simulink model "lab5_2"  (R2020b)
settings: Solver=VariableStepAuto  StartTime=0.0  StopTime=60  RelTol=1e-3
model workspace (MAT data in the model file):
  Kf = 100
  Kp = 100
  x = Simulink.Parameter
  x.Value = 0
  x.DataType = 'auto'
  x.Dimensions = [1 1]
  y = Simulink.Parameter
  y.Value = 1
  y.DataType = 'auto'
  y.Dimensions = [1 1]
settings Model: Creator=Dexp  LastModifiedBy=takem

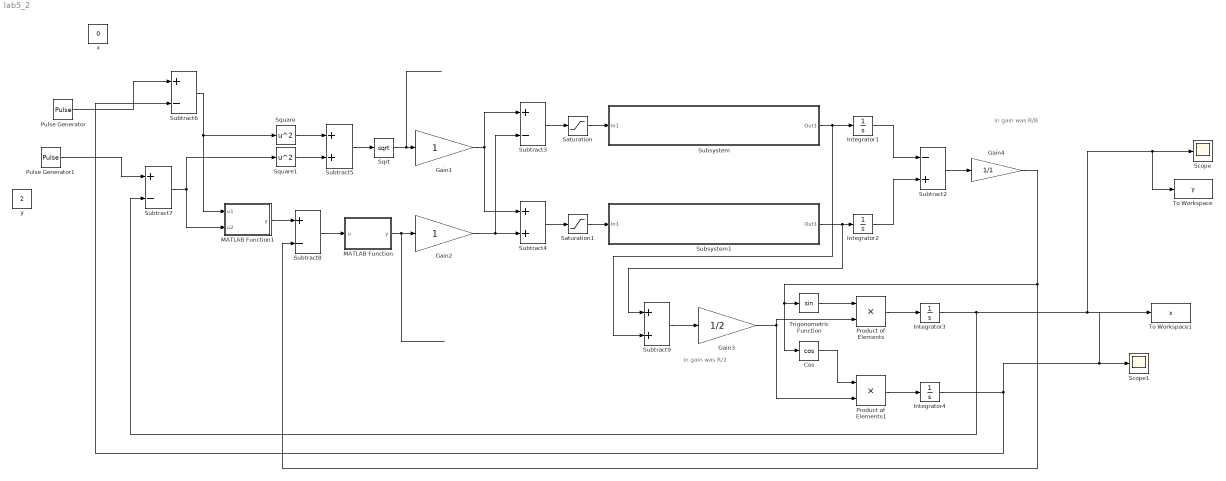
== system lab5_2 ==
  note: in gain was
      | R/B
  note: in gain was
      | R/2
  Cos : Trigonometry  Operator=cos
  Gain1 : Gain
  Gain2 : Gain
  Gain3 : Gain  Gain=1/2
  Gain4 : Gain  Gain=1/1
  Integrator{1..4} (4 alike) : Integrator
  MATLAB Function : MATLAB Function  TreatAsAtomicUnit=on
  MATLAB Function1 : MATLAB Function  TreatAsAtomicUnit=on
  Product of Elements : Product  Inputs=**
  Product of Elements1 : Product  Inputs=**
  Pulse Generator : DiscretePulseGenerator  PulseType=Time based  Period=60  PulseWidth=5  PhaseDelay=30
  Pulse Generator1 : DiscretePulseGenerator  PulseType=Time based  Amplitude=0.5  Period=60  PulseWidth=5  PhaseDelay=60  VectorParams1D=off
  Saturation : Saturate  UpperLimit=100  LowerLimit=-100
  Saturation1 : Saturate  UpperLimit=100  LowerLimit=-100
  Scope : Scope
  Scope1 : Scope
  Sqrt : Sqrt  SaturateOnIntegerOverflow=on
  Square : Math  Operator=square  SaturateOnIntegerOverflow=on
  Square1 : Math  Operator=square  SaturateOnIntegerOverflow=on
  Subsystem : Subsystem
  Subsystem1 : Subsystem
  Subtract2 : Sum  Inputs=-+
  Subtract{3,6..8} (4 alike) : Sum  Inputs=+-
  Subtract4 : Sum
  Subtract5 : Sum
  Subtract9 : Sum
  To Workspace : ToWorkspace  VariableName=y  SampleTime=-1
  To Workspace1 : ToWorkspace  VariableName=x  SampleTime=-1
  Trigonometric Function : Trigonometry
  x : Constant  Value=0
  y : Constant  Value=2
  wires:
  Integrator1/1 -> Subtract2/1
  Saturation/1 -> Subsystem/1(In1)
  Subsystem/1(Out1) -> Subtract9/2, Integrator1/1
  Subsystem1/1(Out1) -> Subtract9/1, Integrator2/1
  Integrator2/1 -> Subtract2/2
  Subtract2/1 -> Gain4/1
  Saturation1/1 -> Subsystem1/1(In1)
  Subtract3/1 -> Saturation/1
  Subtract4/1 -> Saturation1/1
  Subtract5/1 -> Sqrt/1
  Sqrt/1 -> Gain1/1
  Gain1/1 -> Subtract3/1, Subtract4/1
  Gain2/1 -> Subtract3/2, Subtract4/2
  Square/1 -> Subtract5/1
  Square1/1 -> Subtract5/2
  MATLAB Function/1(y) -> Gain2/1
  Subtract8/1 -> MATLAB Function/1(u)
  MATLAB Function1/1(y) -> Subtract8/1
  Subtract6/1 -> MATLAB Function1/1(u1), Square/1
  Subtract7/1 -> MATLAB Function1/2(u2), Square1/1
  Subtract9/1 -> Gain3/1
  Gain4/1 -> Cos/1, Trigonometric Function/1, Subtract8/2
  Trigonometric Function/1 -> Product of Elements/1
  Cos/1 -> Product of Elements1/1
  Gain3/1 -> Product of Elements/2, Product of Elements1/2
  Product of Elements1/1 -> Integrator4/1
  Product of Elements/1 -> Integrator3/1
  Integrator3/1 -> Subtract7/2, To Workspace/1, Scope/1
  Integrator4/1 -> To Workspace1/1, Scope1/1, Subtract6/2
  Pulse Generator/1 -> Subtract6/1
  Pulse Generator1/1 -> Subtract7/1

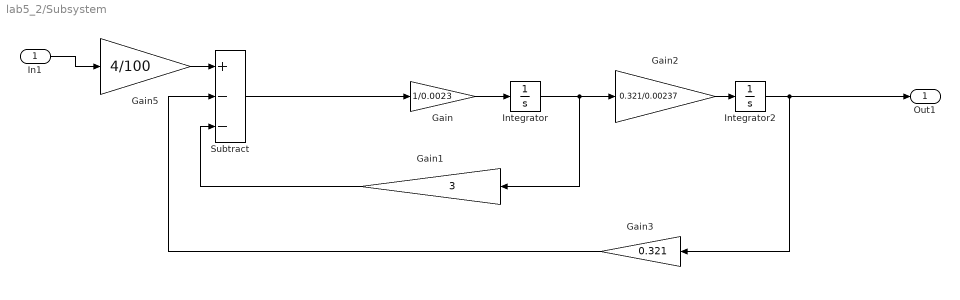
== system lab5_2/Subsystem ==
  In1 : Inport
  Gain : Gain  Gain=1/0.0023
  Gain1 : Gain  Gain=3
  Gain2 : Gain  Gain=0.321/0.00237
  Gain3 : Gain  Gain=0.321
  Gain5 : Gain  Gain=4/100
  Integrator : Integrator
  Integrator2 : Integrator
  Subtract : Sum  Inputs=+--
  Out1 : Outport
  wires:
  Gain5/1 -> Subtract/1
  Gain2/1 -> Integrator2/1
  Integrator/1 -> Gain2/1, Gain1/1
  Gain3/1 -> Subtract/2
  Gain/1 -> Integrator/1
  Integrator2/1 -> Out1/1, Gain3/1
  Subtract/1 -> Gain/1
  Gain1/1 -> Subtract/3
  In1/1 -> Gain5/1

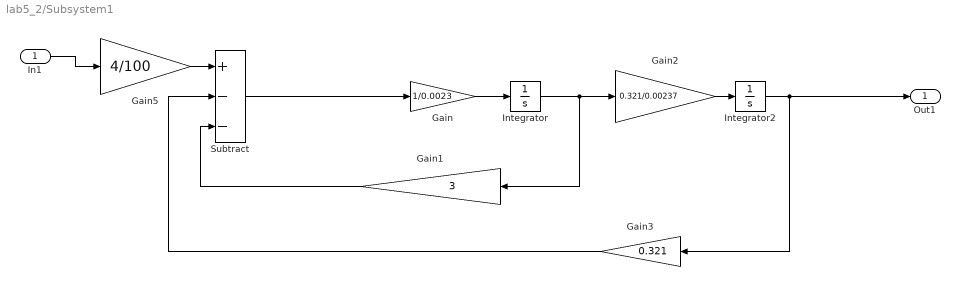
== system lab5_2/Subsystem1 ==
  In1 : Inport
  Gain : Gain  Gain=1/0.0023
  Gain1 : Gain  Gain=3
  Gain2 : Gain  Gain=0.321/0.00237
  Gain3 : Gain  Gain=0.321
  Gain5 : Gain  Gain=4/100
  Integrator : Integrator
  Integrator2 : Integrator
  Subtract : Sum  Inputs=+--
  Out1 : Outport
  wires:
  Gain5/1 -> Subtract/1
  Gain2/1 -> Integrator2/1
  Integrator/1 -> Gain2/1, Gain1/1
  Gain3/1 -> Subtract/2
  Gain/1 -> Integrator/1
  Integrator2/1 -> Out1/1, Gain3/1
  Subtract/1 -> Gain/1
  Gain1/1 -> Subtract/3
  In1/1 -> Gain5/1

== matlab function lab5_2/MATLAB Function ==
  data: u input; y output
function y = fcn(u)
if abs(u)>pi
    y = u - sign(u)*2*pi;
else
    y = u;
end

== matlab function lab5_2/MATLAB Function1 ==
  data: u1 input; y output; u2 input
function y = fcn(u1, u2)
y = atan2(u2, u1);
end
